simulink model "test_model1"  (Simulink 7.0)
settings: Solver=FixedStepDiscrete  StartTime=0.0  StopTime=10.0  FixedStep=0.01  RelTol=1e-3
libraries: Mercury x3
settings Model: Creator=tmaierko  LastModifiedBy=tmaierko
settings OptimizationCC: InlineParams=on  InlineInvariantSignals=on  OptimizeModelRefInitCode=on  LifeSpan=1
settings DebuggingCC: SaveWithParameterizedLinksMsg=none
settings RTWCC: SystemTargetFile=ert.tlc  GenCodeOnly=on  TemplateMakefile=ert_default_tmf  Description=Real-Time Workshop Embedded Coder (no auto configuration)  GenerateReport=on  ProcessScript=ert_make_rtw_hook  IncludeHyperlinkInReport=on  LaunchReport=on
settings CodeAppCC: ForceParamTrailComments=on  IgnoreCustomStorageClasses=off  SimulinkDataObjDesc=on  InsertBlockDesc=on
settings ERTTargetCC: GenFloatMathFcnCalls=ANSI_C  GenerateSampleERTMain=on  SupportAbsoluteTime=off  SupportNonFinite=off  SupportComplex=off  ERTCustomFileTemplate=example_file_process.tlc

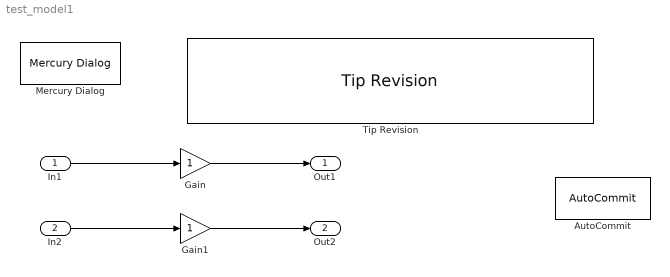
== system test_model1 ==
  In1 : Inport  OutDataType=fixdt(1, 16)  OutScaling=2^0
  In2 : Inport  Port=2  OutDataType=fixdt(1, 16)  OutScaling=2^0
  AutoCommit : Mercury/AutoCommit  SystemSampleTime=-1  ShowInLibBrowser=0
  Gain : Gain  ParameterDataType=fixdt(1, 16)  ParameterScaling=2^0  OutDataType=fixdt(1, 16)  OutScaling=2^0
  Gain1 : Gain  ParameterDataType=fixdt(1, 16)  ParameterScaling=2^0  OutDataType=fixdt(1, 16)  OutScaling=2^0
  Mercury Dialog : Mercury/Mercury Dialog  SystemSampleTime=-1  ShowInLibBrowser=0
  Tip Revision : Mercury/Tip Revision  SystemSampleTime=-1  tip=|  ShowInLibBrowser=0
      | changeset:   124:557440dd8f99
      | tag:         tip
      | user:        Thomas Maier-Komor <thomas.maier-komor@mathworks.de>
      | date:        Tue Jun 15 10:58:45 2010 +0200
      | summary:     updates to comply with requirements of MatlabCentral
  Out1 : Outport  OutDataType=fixdt(1, 16)  OutScaling=2^0
  Out2 : Outport  Port=2  OutDataType=fixdt(1, 16)  OutScaling=2^0
  wires:
  Gain/1 -> Out1/1
  In1/1 -> Gain/1
  Gain1/1 -> Out2/1
  In2/1 -> Gain1/1
